simulink model "RobotModel"  (R2020b)
settings: Solver=ode23s  StartTime=tSim(1)  StopTime=tSim(end)  FixedStep=tStep  RelTol=1e-3  EnableMultiTasking=on
values from neighbouring files (symbols this model uses):
  A = [0,0,0,1,0,0;0,0,0,0,1,0;0,0,0,0,0,1;0,981/2480,0,-27/3100,0,0;0,0,-1635,0,0,0;0,-42183/6200,0,9/1550,0,0]    [DeriveCoefficients.m]    (also in InitController.m; SystemAnalysis.m = subs(A_,{phi,z,xd,phid,zd},{0,0,0,0,0}))
  B = [0,0;0,0;0,0;37500/1271,0;0,10000/3;-25000/1271,0]    [DeriveCoefficients.m]    (also in InitController.m; SystemAnalysis.m = subs(B_,{phi,z,xd,phid,zd},{0,0,0,0,0}))
  C = [1,0,0,0,0,0;0,1,0,0,0,0;0,0,1,0,0,0]    [DeriveCoefficients.m]    (also in InitController.m; SystemAnalysis.m = subs(C_,{phi,z,xd,phid,zd},{0,0,0,0,0}))
  Disturbance = 0.1    [SimulateRobot.m]
  g = 9.81    [SimulateRobot.m]    (also in SystemAnalysis.m)
  IC = [xStart; phiStart; zStart; x_dotStart; phi_dotStart; z_dotStart]    [SimulateRobot.m]
  k_r = 7.2e-3    (= 0.0072)    [SimulateRobot.m]
  L = L'    [InitController.m]
  l_S = 5    [SimulateRobot.m]
  l_W = 0.6    [SimulateRobot.m]
  m_B = 0.05    [SimulateRobot.m]
  m_R = 0.8    [SimulateRobot.m]
  m_W = 0.01    [SimulateRobot.m]
  P_max = wM_max*M_max    (= 3.56)    [SimulateRobot.m]
  phi_max = pi/2    (= 1.57079632679)    [SimulateRobot.m]
  r_R = 0.041    [SimulateRobot.m]
  ricatti_controller = lqr(A,B,Q,S)    [InitController.m]
  u_max = 100    [SimulateRobot.m]
  xStart = 0.25    [SimulateRobot.m]
libraries: simulink x1
settings Model: Creator=loehning  LastModifiedBy=klaus
settings DataIOCC: SaveFormat=Array  SignalLoggingSaveFormat=ModelDataLogs  ReturnWorkspaceOutputs=off
settings OptimizationCC: ExpressionDepthLimit=2147483647  LifeSpan=inf
settings DebuggingCC: UnderspecifiedInitializationDetection=Classic  MergeDetectMultiDrivingBlocksExec=none  SolverPrmCheckMsg=warning  FcnCallInpInsideContextMsg=warning  StateNameClashWarn=warning  PregeneratedLibrarySubsystemCodeDiagnostic=none  SFUnexpectedBacktrackingDiag=warning  SFNoUnconditionalDefaultTransitionDiag=warning  SFExecutionAtInitializationDiag=none  ArithmeticOperatorsInVariantConditions=warning
settings HardwareCC: ProdBitPerPointer=32  ProdBitPerSizeT=32  ProdBitPerPtrDiffT=32  ProdLargestAtomicFloat=None  ProdIntDivRoundTo=Undefined  ProdEndianess=Unspecified  ProdWordSize=32  ProdHWDeviceType=32-bit Generic
settings ModelReferenceCC: PropagateSignalLabelsOutOfModel=off
settings SFSimCC: SimUseLocalCustomCode=off  CustomCodeUndefinedFunction=UseInterfaceOnly
settings RTWCC: RTWUseLocalCustomCode=off
settings CodeAppCC: StateflowObjectComments=on
settings GRTTargetCC: TargetLangStandard=C89/C90 (ANSI)  CombineOutputUpdateFcns=off  GRTInterface=on
settings ConfigComp: CovMetricSettings=dw  CovSaveCumulativeToWorkspaceVar=on  CovSaveSingleToWorkspaceVar=on  CovExternalEMLEnable=off  CovSFcnEnable=off

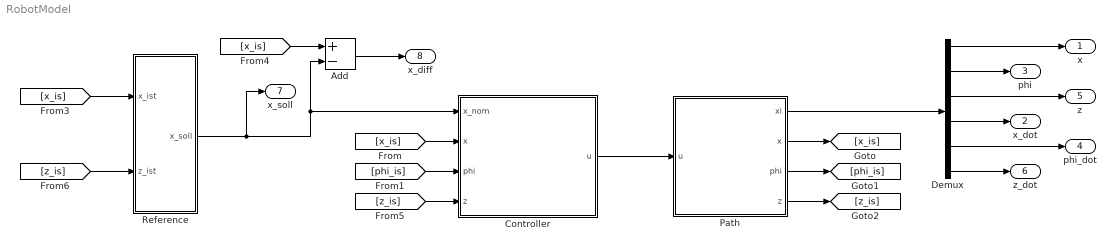
== system RobotModel ==
  Add : Sum  Inputs=+-
  Controller : Subsystem
  Demux : Demux  Outputs=6
  Path : Subsystem
  "Reference " : Subsystem
  x : Outport  VectorParamsAs1DForOutWhenUnconnected=off
  x_dot : Outport  Port=2  VectorParamsAs1DForOutWhenUnconnected=off
  phi : Outport  Port=3  VectorParamsAs1DForOutWhenUnconnected=off
  phi_dot : Outport  Port=4  VectorParamsAs1DForOutWhenUnconnected=off
  z : Outport  Port=5  VectorParamsAs1DForOutWhenUnconnected=off
  z_dot : Outport  Port=6  VectorParamsAs1DForOutWhenUnconnected=off
  x_soll : Outport  Port=7  VectorParamsAs1DForOutWhenUnconnected=off
  x_diff : Outport  Port=8  VectorParamsAs1DForOutWhenUnconnected=off
  wires:
  Path/1(xi) -> Demux/1
  "Reference "/1("x_soll ") -> x_soll/1, Add/2, Controller/1("x_nom ")
  Add/1 -> x_diff/1
  Path/2(x) -> [x_is]
  Path/3(phi) -> [phi_is]
  [x_is] -> Controller/2(x)
  [phi_is] -> Controller/3(phi)
  [z_is] -> "Reference "/2(z_ist)
  [x_is] -> "Reference "/1(x_ist)
  [x_is] -> Add/1
  Path/4(z) -> [z_is]
  [z_is] -> Controller/4(z)
  Demux/1 -> x/1
  Demux/2 -> phi/1
  Demux/3 -> z/1
  Demux/4 -> x_dot/1
  Demux/6 -> z_dot/1
  Demux/5 -> phi_dot/1
  Controller/1(u) -> Path/1("u ")

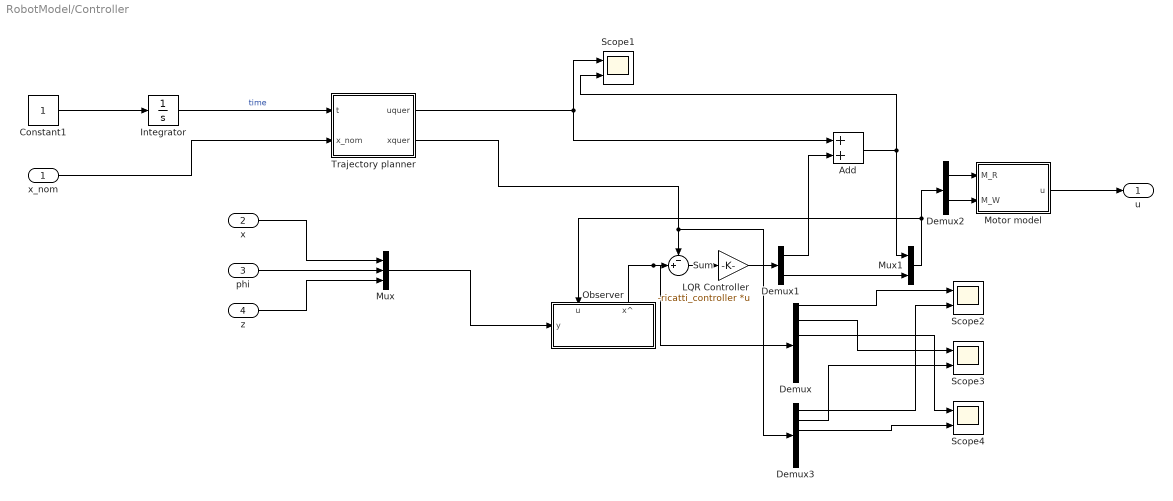
== system RobotModel/Controller ==
  "x_nom " : Inport
  x : Inport  Port=2
  phi : Inport  Port=3
  z : Inport  Port=4
  Add : Sum
  Constant1 : Constant
  Demux : Demux  Outputs=6
  Demux1 : Demux  Outputs=2
  Demux2 : Demux  Outputs=2
  Demux3 : Demux  Outputs=6
  Integrator : Integrator
  LQR Controller : Gain  Gain=-ricatti_controller  Multiplication=Matrix(K*u)
  Motor model : MATLAB Function  TreatAsAtomicUnit=on
  Mux : Mux  Inputs=3
  Mux1 : Mux  Inputs=2
  Observer : Subsystem
      settings: PortSchema="{\"entries\":[{\"content\":{\"sides\":[{\"content\":{\"connectorIds\":[]},\"type\":\"ConnectorPlacement.EquallySpacedRectSide\",\"uuid\":\"22a8423b-4933-4d51-83bb-0edf08131761\"},{\"content\":{\"connectorIds\":[\"In2\"],\"side\":\"RIGHT\"},\"type\":\"ConnectorPlacement.EquallySpacedRectSide\",\"uuid\":\"5b9d6d1b-98ab-4219-9af7-7fee9c92a51b\"},{\"content\":{\"connectorIds\":[],\"side\":\"TOP\"},\"type\":\"ConnectorPlacement.EquallySpacedRectSide\",\"uuid\":\"36e21f0c-31ec-4f4a-8214-47493b03beb7\"},{\"content\":{\"connectorIds\":[\"Out1\",\"In1\"],\"side\":\"BOTTOM\"},\"type\":\"ConnectorPlacement.EquallySpacedRectSide\",\"uuid\":\"16be921e-dd10-4af0-8f26-903c539fc89e\"},{\"content\":{\"connectorIds\":[],\"side\":\"HIDDEN\"},\"type\":\"ConnectorPlacement.EquallySpacedRectSide\",\"uuid\":\"78228177-2ce9-4310-9ad2-dd2810dc3955\"}]},\"type\":\"ConnectorPlacement.EquallySpacedConnector\",\"uuid\":\"efa65d2b-dbcd-4652-bcaa-bff7c8215a9d\"}],\"packageUris\":[\"http://schema.mathworks.com/mf0/Connector/R2020b\"],\"version\":\"1.0\"}"
  Scope{1..4} (4 alike) : Scope  NumInputPorts=2
  Sum : Sum  Inputs=-+|
  Trajectory planner : Subsystem
  u : Outport  VectorParamsAs1DForOutWhenUnconnected=off
  wires:
  Motor model/1(u) -> u/1
  Trajectory planner/1(uquer) -> Scope1/1, Add/1
  Add/1 -> Mux1/1, Scope1/2
  Constant1/1 -> Integrator/1
  Integrator/1 -> Trajectory planner/1(t)  "time"
  Trajectory planner/2(xquer) -> Demux3/1, Sum/1
  "x_nom "/1 -> Trajectory planner/2(x_nom)
  Mux1/1 -> Demux2/1, Observer/1(u)
  phi/1 -> Mux/2
  Mux/1 -> Observer/2(y)
  z/1 -> Mux/3
  x/1 -> Mux/1
  LQR Controller/1 -> Demux1/1
  Demux1/1 -> Add/2
  Demux1/2 -> Mux1/2
  Demux2/1 -> Motor model/1(M_R)
  Demux2/2 -> Motor model/2(M_W)
  Sum/1 -> LQR Controller/1
  Observer/1(x^) -> Demux/1, Sum/2
  Demux/1 -> Scope2/1
  Demux3/1 -> Scope2/2
  Demux/2 -> Scope3/1
  Demux3/2 -> Scope3/2
  Demux/3 -> Scope4/1
  Demux3/3 -> Scope4/2

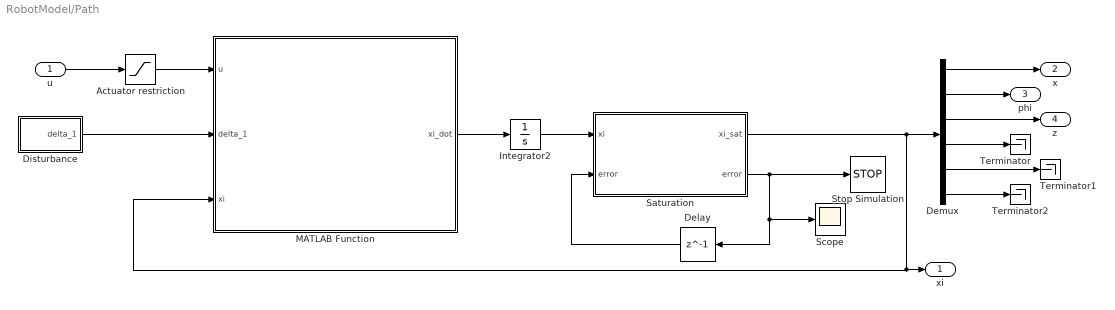
== system RobotModel/Path ==
  "u " : Inport
  Actuator restriction : Saturate  UpperLimit=[u_max;u_max]  LowerLimit=-[u_max;u_max]
  Delay : Delay  DelayLength=1  InitialCondition=0
  Demux : Demux  Outputs=6
  Disturbance : Subsystem
  Integrator2 : Integrator  InitialCondition=IC
  MATLAB Function : MATLAB Function  TreatAsAtomicUnit=on
  "Saturation " : MATLAB Function  TreatAsAtomicUnit=on
  Scope : Scope
  Stop Simulation : Stop
  Terminator : Terminator
  Terminator1 : Terminator
  Terminator2 : Terminator
  xi : Outport  VectorParamsAs1DForOutWhenUnconnected=off
  x : Outport  Port=2  VectorParamsAs1DForOutWhenUnconnected=off
  phi : Outport  Port=3  VectorParamsAs1DForOutWhenUnconnected=off
  z : Outport  Port=4  VectorParamsAs1DForOutWhenUnconnected=off
  wires:
  MATLAB Function/1(xi_dot) -> Integrator2/1
  Delay/1 -> "Saturation "/2("error ")
  "Saturation "/2(error) -> Stop Simulation/1, Scope/1, Delay/1
  Disturbance/1("delta_1 ") -> MATLAB Function/2(delta_1)
  Integrator2/1 -> "Saturation "/1(xi)
  Actuator restriction/1 -> MATLAB Function/1(u)
  Demux/1 -> x/1
  Demux/2 -> phi/1
  Demux/3 -> z/1
  Demux/4 -> Terminator/1
  Demux/5 -> Terminator1/1
  Demux/6 -> Terminator2/1
  "Saturation "/1(xi_sat) -> Demux/1, xi/1, MATLAB Function/3(xi)
  "u "/1 -> Actuator restriction/1

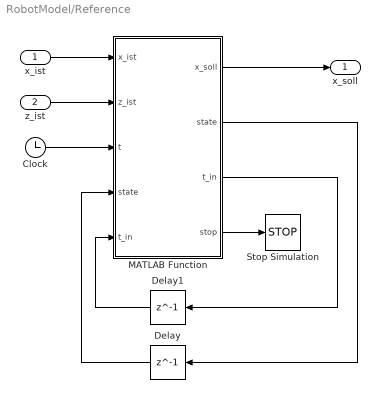
== system RobotModel/Reference  ==
  x_ist : Inport
  z_ist : Inport  Port=2
  Clock : Clock
  Delay : Delay  DelayLength=1  InitialCondition=1
  Delay1 : Delay  DelayLength=1
  MATLAB Function : MATLAB Function  TreatAsAtomicUnit=on
  Stop Simulation : Stop
  "x_soll " : Outport  VectorParamsAs1DForOutWhenUnconnected=off
  wires:
  MATLAB Function/2(state) -> Delay/1
  Delay/1 -> MATLAB Function/4("state ")
  Clock/1 -> MATLAB Function/3(t)
  x_ist/1 -> MATLAB Function/1(x_ist)
  z_ist/1 -> MATLAB Function/2(z_ist)
  MATLAB Function/1(x_soll) -> "x_soll "/1
  MATLAB Function/3(t_in) -> Delay1/1
  Delay1/1 -> MATLAB Function/5("t_in ")
  MATLAB Function/4(stop) -> Stop Simulation/1

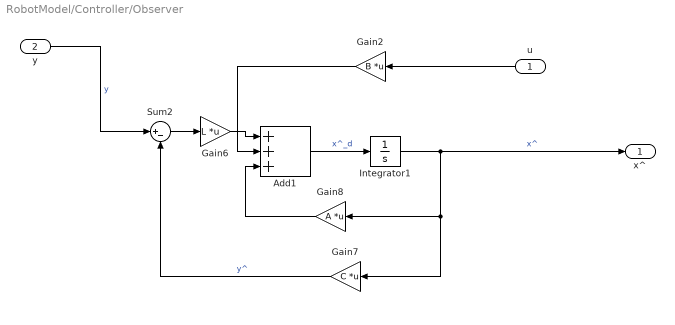
== system RobotModel/Controller/Observer ==
  u : Inport
  y : Inport  Port=2
  Add1 : Sum  Inputs=+++
  Gain2 : Gain  Gain=B  Multiplication=Matrix(K*u)
  Gain6 : Gain  Gain=L  Multiplication=Matrix(K*u)
  Gain7 : Gain  Gain=C  Multiplication=Matrix(K*u)
  Gain8 : Gain  Gain=A  Multiplication=Matrix(K*u)
  Integrator1 : Integrator  InitialCondition=IC
  Sum2 : Sum  Inputs=|+-
  x^ : Outport
  wires:
  Gain2/1 -> Add1/2
  u/1 -> Gain2/1
  Integrator1/1 -> x^/1, Gain7/1, Gain8/1  "x^"
  Gain7/1 -> Sum2/2  "y^"
  y/1 -> Sum2/1  "y"
  Gain6/1 -> Add1/1
  Sum2/1 -> Gain6/1
  Add1/1 -> Integrator1/1  "x^_d"
  Gain8/1 -> Add1/3

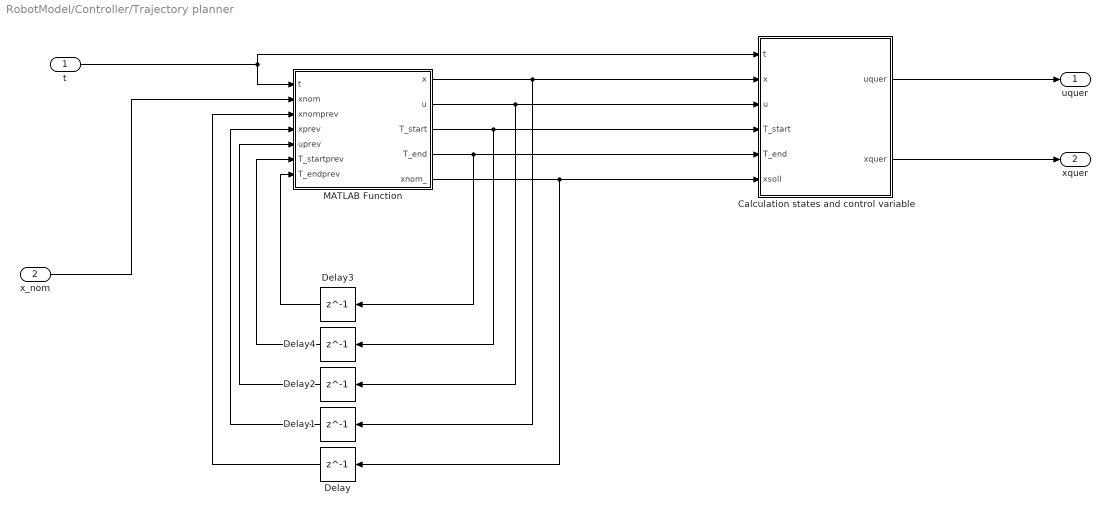
== system RobotModel/Controller/Trajectory planner ==
  t : Inport
  x_nom : Inport  Port=2
  Calculation states and control variable : MATLAB Function  TreatAsAtomicUnit=on
  Delay : Delay  DelayLength=1  InitialCondition=xStart
  Delay{1..4} (4 alike) : Delay  DelayLength=1
  MATLAB Function : MATLAB Function  TreatAsAtomicUnit=on
  uquer : Outport
  xquer : Outport  Port=2
  wires:
  MATLAB Function/1(x) -> Delay1/1, Calculation states and control variable/2(x)
  Delay3/1 -> MATLAB Function/7(T_endprev)
  MATLAB Function/4(T_end) -> Delay3/1, Calculation states and control variable/5(T_end)
  MATLAB Function/2(u) -> Delay2/1, Calculation states and control variable/3(u)
  Delay4/1 -> MATLAB Function/6(T_startprev)
  t/1 -> Calculation states and control variable/1(t), MATLAB Function/1(t)
  Delay1/1 -> MATLAB Function/4(xprev)
  Delay/1 -> MATLAB Function/3(xnomprev)
  MATLAB Function/3(T_start) -> Delay4/1, Calculation states and control variable/4(T_start)
  x_nom/1 -> MATLAB Function/2(xnom)
  Delay2/1 -> MATLAB Function/5(uprev)
  MATLAB Function/5(xnom_) -> Calculation states and control variable/6(xsoll), Delay/1
  Calculation states and control variable/2(xquer) -> xquer/1
  Calculation states and control variable/1(uquer) -> uquer/1

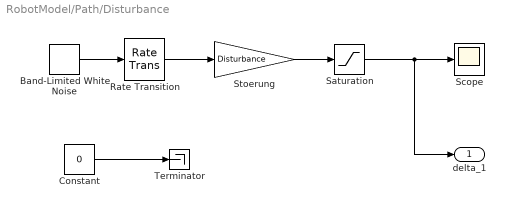
== system RobotModel/Path/Disturbance ==
  Band-Limited White Noise : simulink/Sources/Band-Limited White Noise  Cov=disturbanceNoisePower  Ts=0.025  seed=disturbanceSeed_1
  Constant : Constant  Value=0
  Rate Transition : RateTransition
  Saturation : Saturate  UpperLimit=3  LowerLimit=-3
  Scope : Scope
  Stoerung : Gain  Gain=Disturbance
  Terminator : Terminator
  "delta_1 " : Outport  VectorParamsAs1DForOutWhenUnconnected=off
  wires:
  Band-Limited White Noise/1 -> Rate Transition/1
  Rate Transition/1 -> Stoerung/1
  Stoerung/1 -> Saturation/1
  Saturation/1 -> "delta_1 "/1, Scope/1
  Constant/1 -> Terminator/1

== matlab function RobotModel/Controller/Trajectory planner/Calculation states and control variable ==
  data: t input; uquer output; xquer output; x input; u input; T_start input; T_end input; xsoll input
function [uquer, xquer] = fcn(t, x, u, T_start, T_end, xsoll)
  if t<T_end && size(x,2) == 68 && size(u,2) == 12 
      xquer = [x(1)*(t-T_start)^13+x(2)*(t-T_start)^12+x(3)*(t-T_start)^11+x(4)*(t-T_start)^10+x(5)*(t-T_start)^9+x(6)*(t-T_start)^8+x(7)*(t-T_start)^7+x(8)*(t-T_start)^6+x(9)*(t-T_start)^5+x(10)*(t-T_start)^4+x(11)*(t-T_start)^3+x(12)*(t-T_start)^2+x(13);...
      x(14)*(t-T_start)^12+x(15)*(t-T_start)^11+x(16)*(t-T_start)^10+x(17)*(t-T_start)^9+x(18)*(t-T_start)^8+x(19)*(t-T_start)^7+x(20)*(t-T_start)^6+x(21)*(t-T_start)^5+x(22)*(t-T_start)^4+x(23)*(t-T_start)^3+x(24)*(t-T_start)^2;...
      x(25)*(t-T_start)^12+x(26)*(t-T_start)^11+x(27)*(t-T_start)^10+x(28)*(t-T_start)^9+x(29)*(t-T_start)^8+x(30)*(t-T_start)^7+x(31)*(t-T_start)^6+x(32)*(t-T_start)^5+x(33)*(t-T_start)^4+x(34)*(t-T_start)^3+x(35)*(t-T_start)^2;...
      x(36)*(t-T_start)^12+x(37)*(t-T_start)^11+x(38)*(t-T_start)^10+x(39)*(t-T_start)^9+x(40)*(t-T_start)^8+x(41)*(t-T_start)^7+x(42)*(t-T_start)^6+x(43)*(t-T_start)^5+x(44)*(t-T_start)^4+x(45)*(t-T_start)^3+x(46)*(t-T_start)^2;...
      x(47)*(t-T_start)^12+x(48)*(t-T_start)^11+x(49)*(t-T_start)^10+x(50)*(t-T_start)^9+x(51)*(t-T_start)^8+x(52)*(t-T_start)^7+x(53)*(t-T_start)^6+x(54)*(t-T_start)^5+x(55)*(t-T_start)^4+x(56)*(t-T_start)^3+x(57)*(t-T_start)^2;...
      x(58)*(t-T_start)^12+x(59)*(t-T_start)^11+x(60)*(t-T_start)^10+x(61)*(t-T_start)^9+x(62)*(t-T_start)^8+x(63)*(t-T_start)^7+x(64)*(t-T_start)^6+x(65)*(t-T_start)^5+x(66)*(t-T_start)^4+x(67)*(t-T_start)^3+x(68)*(t-T_start)^2];
      uquer = u(1)*(t-T_start)^12+u(2)*(t-T_start)^11+u(3)*(t-T_start)^10+u(4)*(t-T_start)^9+u(5)*(t-T_start)^8+u(6)*(t-T_start)^7+u(7)*(t-T_start)^6+u(8)*(t-T_start)^5+u(9)*(t-T_start)^4+u(10)*(t-T_start)^3+u(11)*(t-T_start)^2+u(12)*(t-T_start);
  else
      xquer = [xsoll;0;0;0;0;0];      
      uquer = 0;
  end  
end

== matlab function RobotModel/Controller/Trajectory planner/MATLAB Function ==
  data: x output; t input; xnom input; u output; xnomprev input; T_start output; T_end output; xnom_ output; xprev input; uprev input; T_startprev input; T_endprev input
function [x, u, T_start, T_end, xnom_] = fcn(t, xnom, xnomprev, xprev, uprev, T_startprev, T_endprev)
    if xnom ~= xnomprev
        w0 = xnomprev;
        wT = xnom;
        order = [12,11,10,9,8,7,6,5,4,3,2,1];
        T_end = abs(w0-wT)/0.7;
        if T_end<1
            T_end=1;
        end
        u1 = [(1011384551389116279375*(w0 - wT))/(36893488147419103232*T_end^7), (1092295315500245581725*(w0 - wT))/(9149585060559937601536*T_end^7) - (21239075579171441866875*(w0 - wT))/(36893488147419103232*T_end^8), (35398459298619069778125*(w0 - wT))/(9223372036854775808*T_end^9) - (7646067208501719072075*(w0 - wT))/(4574792530279968800768*T_end^8) - (142538111831879000698793027470149375*(w0 - wT))/(6901746346790563787434755862277025452451108972170386555162524223799296*T_end^7), (2993300348469459014674653576873136875*(w0 - wT))/(13803492693581127574869511724554050904902217944340773110325048447598592*T_end^8) + (38230336042508595360375*(w0 - wT))/(4574792530279968800768*T_end^9) - (106195377895857209334375*(w0 - wT))/(9223372036854775808*T_end^10), (318586133687571628003125*(w0 - wT))/(18446744073709551616*T_end^11) - (2993300348469459014674653576873136875*(w0 - wT))/(3450873173395281893717377931138512726225554486085193277581262111899648*T_end^9) - (22938201625505157216225*(w0 - wT))/(1143698132569992200192*T_end^10) - (51542850267891542935087149177365625*(w0 - wT))/(20282409603651670423947251286016*T_end^7), (360799951875240800545610044241559375*(w0 - wT))/(20282409603651670423947251286016*T_end^8) - (36823171168130880507853335496664625*(w0 - wT))/(10384593717069655257060992658440192*T_end^7) + (2993300348469459014674653576873136875*(w0 - wT))/(1725436586697640946858688965569256363112777243042596638790631055949824*T_end^10) + (114691008127525786081125*(w0 - wT))/(4574792530279968800768*T_end^11) - (233629831370885860535625*(w0 - wT))/(18446744073709551616*T_end^12), (110469513504392641523560006489993875*(w0 - wT))/(5192296858534827628530496329220096*T_end^8) - (257714251339457714675435745886828125*(w0 - wT))/(5070602400912917605986812821504*T_end^9) - (6414215032434555031445686236156721875*(w0 - wT))/(3450873173395281893717377931138512726225554486085193277581262111899648*T_end^11) - (36045745411508104196925*(w0 - wT))/(2287396265139984400384*T_end^12) + (33375690195840837219375*(w0 - wT))/(9223372036854775808*T_end^13), (773142754018373144026307237660484375*(w0 - wT))/(10141204801825835211973625643008*T_end^10) - (552347567521963207617800032449969375*(w0 - wT))/(10384593717069655257060992658440192*T_end^9) + (14111273071356021069180509719544788125*(w0 - wT))/(13803492693581127574869511724554050904902217944340773110325048447598592*T_end^12) + (36045745411508104196925*(w0 - wT))/(9149585060559937601536*T_end^13), (184115855840654402539266677483323125*(w0 - wT))/(2596148429267413814265248164610048*T_end^10) - (1288571256697288573377178729434140625*(w0 - wT))/(20282409603651670423947251286016*T_end^11) - (1567919230150669007686723302171643125*(w0 - wT))/(6901746346790563787434755862277025452451108972170386555162524223799296*T_end^13), (566971352946806972285958640951021875*(w0 - wT))/(20282409603651670423947251286016*T_end^12) - (552347567521963207617800032449969375*(w0 - wT))/(10384593717069655257060992658440192*T_end^11), (110469513504392641523560006489993875*(w0 - wT))/(5192296858534827628530496329220096*T_end^12) - (51542850267891542935087149177365625*(w0 - wT))/(10141204801825835211973625643008*T_end^13), -(36823171168130880507853335496664625*(w0 - wT))/(10384593717069655257060992658440192*T_end^13)];
        u = double(u1(order));
        order = [13,12,11,10,9,8,7,6,5,4,3,2,1,24,23,22,21,20,19,18,17,16,15,14,35,34,33,32,31,30,29,28,27,26,25,46,45,44,43,42,41,40,39,38,37,36,57,56,55,54,53,52,51,50,49,48,47,68,67,66,65,64,63,62,61,60,59,58];
        x1 = [w0, -(91300322845796259195*(w0 - wT))/(89202980794122492566142873090593446023921664*T_end^7), (155417816831775633135*(w0 - wT))/(1152921504606846976*T_end^7) + (639102259920573814365*(w0 - wT))/(44601490397061246283071436545296723011960832*T_end^8), - (159970356708403816575*(w0 - wT))/(340282366920938463463374607431768211456*T_end^7) - (3263774153467288295835*(w0 - wT))/(2305843009213693952*T_end^8) - (3195511299602869071825*(w0 - wT))/(44601490397061246283071436545296723011960832*T_end^9), (15686105019335663913*(w0 - wT))/(43556142965880123323311949751266331066368*T_end^7) + (671875498175296029615*(w0 - wT))/(170141183460469231731687303715884105728*T_end^8) + (3263774153467288295835*(w0 - wT))/(576460752303423488*T_end^9) + (1917306779761721443095*(w0 - wT))/(11150372599265311570767859136324180752990208*T_end^10), (21186311244744238593*(w0 - wT))/(696898287454081973172991196020261297061888*T_end^7) - (109802735135349647391*(w0 - wT))/(43556142965880123323311949751266331066368*T_end^8) - (1119792496958826716025*(w0 - wT))/(85070591730234615865843651857942052864*T_end^9) - (3263774153467288295835*(w0 - wT))/(288230376151711744*T_end^10) - (9586533898808607215475*(w0 - wT))/(44601490397061246283071436545296723011960832*T_end^11), (78430525096678319565*(w0 - wT))/(10889035741470030830827987437816582766592*T_end^9) - (63558933734232715779*(w0 - wT))/(348449143727040986586495598010130648530944*T_end^8) - (1716*(w0 - wT))/T_end^7 + (479911070125211449725*(w0 - wT))/(21267647932558653966460912964485513216*T_end^10) + (6993801757429903491075*(w0 - wT))/(576460752303423488*T_end^11) + (3012910653911276553435*(w0 - wT))/(22300745198530623141535718272648361505980416*T_end^12), (9009*(w0 - wT))/T_end^8 + (317794668671163578895*(w0 - wT))/(696898287454081973172991196020261297061888*T_end^9) - (235291575290034958695*(w0 - wT))/(21778071482940061661655974875633165533184*T_end^10) - (7198666051878171745875*(w0 - wT))/(340282366920938463463374607431768211456*T_end^11) - (15386363866345787680365*(w0 - wT))/(2305843009213693952*T_end^12) - (3012910653911276553435*(w0 - wT))/(89202980794122492566142873090593446023921664*T_end^13), (392152625483391597825*(w0 - wT))/(43556142965880123323311949751266331066368*T_end^11) - (105931556223721192965*(w0 - wT))/(174224571863520493293247799005065324265472*T_end^10) - (20020*(w0 - wT))/T_end^9 + (1759673923792441982325*(w0 - wT))/(170141183460469231731687303715884105728*T_end^12) + (1709595985149531964485*(w0 - wT))/(1152921504606846976*T_end^13), (24024*(w0 - wT))/T_end^10 + (317794668671163578895*(w0 - wT))/(696898287454081973172991196020261297061888*T_end^11) - (172547155212692303043*(w0 - wT))/(43556142965880123323311949751266331066368*T_end^12) - (351934784758488396465*(w0 - wT))/(170141183460469231731687303715884105728*T_end^13), (15686105019335663913*(w0 - wT))/(21778071482940061661655974875633165533184*T_end^13) - (63558933734232715779*(w0 - wT))/(348449143727040986586495598010130648530944*T_end^12) - (16380*(w0 - wT))/T_end^11, (6006*(w0 - wT))/T_end^12 + (21186311244744238593*(w0 - wT))/(696898287454081973172991196020261297061888*T_end^13), -(924*(w0 - wT))/T_end^13, -(1213230839868007845885*(w0 - wT))/(85070591730234615865843651857942052864*T_end^7), (8492615879076054921195*(w0 - wT))/(42535295865117307932921825928971026432*T_end^8) - (252577308855890773755*(w0 - wT))/(10889035741470030830827987437816582766592*T_end^7), (5304123485973706248855*(w0 - wT))/(21778071482940061661655974875633165533184*T_end^8) - (74318744670378353145*(w0 - wT))/(1393796574908163946345982392040522594123776*T_end^7) - (42463079395380274605975*(w0 - wT))/(42535295865117307932921825928971026432*T_end^9), (800800*(w0 - wT))/(109*T_end^7) + (312138727615589083209*(w0 - wT))/(696898287454081973172991196020261297061888*T_end^8) - (5304123485973706248855*(w0 - wT))/(5444517870735015415413993718908291383296*T_end^9) + (25477847637228164763585*(w0 - wT))/(10633823966279326983230456482242756608*T_end^10), (5304123485973706248855*(w0 - wT))/(2722258935367507707706996859454145691648*T_end^10) - (5605600*(w0 - wT))/(109*T_end^8) - (520231212692648472015*(w0 - wT))/(348449143727040986586495598010130648530944*T_end^9) - (22057997440968149661*(w0 - wT))/(5192296858534827628530496329220096*T_end^7) - (127389238186140823817925*(w0 - wT))/(42535295865117307932921825928971026432*T_end^11), (66173992322904448983*(w0 - wT))/(2596148429267413814265248164610048*T_end^8) + (16016000*(w0 - wT))/(109*T_end^9) + (222956234011135059435*(w0 - wT))/(87112285931760246646623899502532662132736*T_end^10) - (11365978898515084818975*(w0 - wT))/(5444517870735015415413993718908291383296*T_end^11) + (40036617715644258914205*(w0 - wT))/(21267647932558653966460912964485513216*T_end^12), (25005153576733186601745*(w0 - wT))/(21778071482940061661655974875633165533184*T_end^12) - (24024000*(w0 - wT))/(109*T_end^10) - (3344343510167025891525*(w0 - wT))/(1393796574908163946345982392040522594123776*T_end^11) - (330869961614522244915*(w0 - wT))/(5192296858534827628530496329220096*T_end^9) - (40036617715644258914205*(w0 - wT))/(85070591730234615865843651857942052864*T_end^13), (110289987204840748305*(w0 - wT))/(1298074214633706907132624082305024*T_end^10) + (20020000*(w0 - wT))/(109*T_end^11) + (817506191374161884595*(w0 - wT))/(696898287454081973172991196020261297061888*T_end^12) - (2778350397414798511305*(w0 - wT))/(10889035741470030830827987437816582766592*T_end^13), - (330869961614522244915*(w0 - wT))/(5192296858534827628530496329220096*T_end^11) - (8808800*(w0 - wT))/(109*T_end^12) - (163501238274832376919*(w0 - wT))/(696898287454081973172991196020261297061888*T_end^13), (66173992322904448983*(w0 - wT))/(2596148429267413814265248164610048*T_end^12) + (1601600*(w0 - wT))/(109*T_end^13), -(22057997440968149661*(w0 - wT))/(5192296858534827628530496329220096*T_end^13), (486935055177579913905*(w0 - wT))/(713623846352979940529142984724747568191373312*T_end^7), - (25902969471962598015*(w0 - wT))/(288230376151711744*T_end^7) - (3408545386243059397335*(w0 - wT))/(356811923176489970264571492362373784095686656*T_end^8), (228719772458392380165*(w0 - wT))/(2658455991569831745807614120560689152*T_end^7) + (543962358911214558315*(w0 - wT))/(576460752303423488*T_end^8) + (17042726931215296986675*(w0 - wT))/(356811923176489970264571492362373784095686656*T_end^9), (79978429159320330639*(w0 - wT))/(10889035741470030830827987437816582766592*T_end^7) - (960623044325247996693*(w0 - wT))/(1329227995784915872903807060280344576*T_end^8) - (543962358911214558315*(w0 - wT))/(144115188075855872*T_end^9) - (10225636158729178192005*(w0 - wT))/(89202980794122492566142873090593446023921664*T_end^10), (1601038407208746661155*(w0 - wT))/(664613997892457936451903530140172288*T_end^9) - (559849004115242314473*(w0 - wT))/(10889035741470030830827987437816582766592*T_end^8) - (12046928654849835747*(w0 - wT))/(1393796574908163946345982392040522594123776*T_end^7) + (543962358911214558315*(w0 - wT))/(72057594037927936*T_end^10) + (51128180793645890960025*(w0 - wT))/(356811923176489970264571492362373784095686656*T_end^11), (36140785964549507241*(w0 - wT))/(696898287454081973172991196020261297061888*T_end^8) + (399892145796601653195*(w0 - wT))/(2722258935367507707706996859454145691648*T_end^9) - (686159317375177140495*(w0 - wT))/(166153499473114484112975882535043072*T_end^10) - (1165633626238316910675*(w0 - wT))/(144115188075855872*T_end^11) - (16068856820860137158865*(w0 - wT))/(178405961588244985132285746181186892047843328*T_end^12), (10292389760627657107425*(w0 - wT))/(2658455991569831745807614120560689152*T_end^11) - (1199676437389804959585*(w0 - wT))/(5444517870735015415413993718908291383296*T_end^10) - (180703929822747536205*(w0 - wT))/(1393796574908163946345982392040522594123776*T_end^9) + (2564393977724297203485*(w0 - wT))/(576460752303423488*T_end^12) + (16068856820860137158865*(w0 - wT))/(713623846352979940529142984724747568191373312*T_end^13), (60234643274249178735*(w0 - wT))/(348449143727040986586495598010130648530944*T_end^10) + (1999460728983008265975*(w0 - wT))/(10889035741470030830827987437816582766592*T_end^11) - (2515917497042316181815*(w0 - wT))/(1329227995784915872903807060280344576*T_end^12) - (284932664191588578165*(w0 - wT))/(288230376151711744*T_end^13), (503183499408463236363*(w0 - wT))/(1329227995784915872903807060280344576*T_end^13) - (879762720752523637029*(w0 - wT))/(10889035741470030830827987437816582766592*T_end^12) - (180703929822747536205*(w0 - wT))/(1393796574908163946345982392040522594123776*T_end^11), (36140785964549507241*(w0 - wT))/(696898287454081973172991196020261297061888*T_end^12) + (79978429159320330639*(w0 - wT))/(5444517870735015415413993718908291383296*T_end^13), -(12046928654849835747*(w0 - wT))/(1393796574908163946345982392040522594123776*T_end^13), (466253450495326899405*(w0 - wT))/(1152921504606846976*T_end^7), - (319940713416817227735*(w0 - wT))/(170141183460469231731687303715884105728*T_end^7) - (3263774153467288295835*(w0 - wT))/(576460752303423488*T_end^8), (313722100386713683665*(w0 - wT))/(174224571863520493293247799005065324265472*T_end^7) + (6718754981753161782435*(w0 - wT))/(340282366920938463463374607431768211456*T_end^8) + (16318870767336441479175*(w0 - wT))/(576460752303423488*T_end^9), - (41005763699505051447*(w0 - wT))/(5575186299632655785383929568162090376495104*T_end^7) - (1317632821624197471393*(w0 - wT))/(87112285931760246646623899502532662132736*T_end^8) - (6718754981753161782435*(w0 - wT))/(85070591730234615865843651857942052864*T_end^9) - (9791322460401864887505*(w0 - wT))/(144115188075855872*T_end^10), (287040345896535360129*(w0 - wT))/(5575186299632655785383929568162090376495104*T_end^8) - (12012*(w0 - wT))/T_end^7 + (2196054702706995785655*(w0 - wT))/(43556142965880123323311949751266331066368*T_end^9) + (6718754981753161782435*(w0 - wT))/(42535295865117307932921825928971026432*T_end^10) + (48956612302009324437525*(w0 - wT))/(576460752303423488*T_end^11), (72072*(w0 - wT))/T_end^8 - (205028818497525257235*(w0 - wT))/(1393796574908163946345982392040522594123776*T_end^9) - (941166301160141050995*(w0 - wT))/(10889035741470030830827987437816582766592*T_end^10) - (14397332103756775248075*(w0 - wT))/(85070591730234615865843651857942052864*T_end^11) - (15386363866345787680365*(w0 - wT))/(288230376151711744*T_end^12), (615086455492575771705*(w0 - wT))/(2787593149816327892691964784081045188247552*T_end^10) - (180180*(w0 - wT))/T_end^9 + (14117494517402115764925*(w0 - wT))/(174224571863520493293247799005065324265472*T_end^11) + (31674130628264905545765*(w0 - wT))/(340282366920938463463374607431768211456*T_end^12) + (15386363866345787680365*(w0 - wT))/(1152921504606846976*T_end^13), (240240*(w0 - wT))/T_end^10 - (1025144092487626286175*(w0 - wT))/(5575186299632655785383929568162090376495104*T_end^11) - (3450943104253850520315*(w0 - wT))/(87112285931760246646623899502532662132736*T_end^12) - (3519347847584989505085*(w0 - wT))/(170141183460469231731687303715884105728*T_end^13), (451063400694555565917*(w0 - wT))/(5575186299632655785383929568162090376495104*T_end^12) - (180180*(w0 - wT))/T_end^11 + (690188620850770104063*(w0 - wT))/(87112285931760246646623899502532662132736*T_end^13), (72072*(w0 - wT))/T_end^12 - (41005763699505051447*(w0 - wT))/(2787593149816327892691964784081045188247552*T_end^13), -(12012*(w0 - wT))/T_end^13, (594824777491629980295*(w0 - wT))/(10889035741470030830827987437816582766592*T_end^7), - (297274978681513457625*(w0 - wT))/(1393796574908163946345982392040522594123776*T_end^7) - (4163773442441409862065*(w0 - wT))/(5444517870735015415413993718908291383296*T_end^8), (4004000*(w0 - wT))/(109*T_end^7) + (6242774552311782610125*(w0 - wT))/(2787593149816327892691964784081045188247552*T_end^8) + (20818867212207049310325*(w0 - wT))/(5444517870735015415413993718908291383296*T_end^9), - (36519221481393702051*(w0 - wT))/(1298074214633706907132624082305024*T_end^7) - (33633600*(w0 - wT))/(109*T_end^8) - (6242774552311782610125*(w0 - wT))/(696898287454081973172991196020261297061888*T_end^9) - (12491320327324229586195*(w0 - wT))/(1361129467683753853853498429727072845824*T_end^10), (255634550369755914357*(w0 - wT))/(1298074214633706907132624082305024*T_end^8) - (19616364991367881737*(w0 - wT))/(5316911983139663491615228241121378304*T_end^7) + (112112000*(w0 - wT))/(109*T_end^9) + (6242774552311782610125*(w0 - wT))/(348449143727040986586495598010130648530944*T_end^10) + (62456601636621147930975*(w0 - wT))/(5444517870735015415413993718908291383296*T_end^11), (58849094974103645211*(w0 - wT))/(2658455991569831745807614120560689152*T_end^8) - (182596107406968510255*(w0 - wT))/(324518553658426726783156020576256*T_end^9) - (192192000*(w0 - wT))/(109*T_end^10) - (13377374040668105593125*(w0 - wT))/(696898287454081973172991196020261297061888*T_end^11) - (19629217657223789349735*(w0 - wT))/(2722258935367507707706996859454145691648*T_end^12), (547788322220905530765*(w0 - wT))/(649037107316853453566312041152512*T_end^10) - (294245474870518226055*(w0 - wT))/(5316911983139663491615228241121378304*T_end^9) + (180180000*(w0 - wT))/(109*T_end^11) + (29430222889469832304875*(w0 - wT))/(2787593149816327892691964784081045188247552*T_end^12) + (19629217657223789349735*(w0 - wT))/(10889035741470030830827987437816582766592*T_end^13), (98081824956839408685*(w0 - wT))/(1329227995784915872903807060280344576*T_end^10) - (912980537034842551275*(w0 - wT))/(1298074214633706907132624082305024*T_end^11) - (88088000*(w0 - wT))/(109*T_end^12) - (3270024765496648033875*(w0 - wT))/(1393796574908163946345982392040522594123776*T_end^13), (401711436295330722561*(w0 - wT))/(1298074214633706907132624082305024*T_end^12) - (294245474870518226055*(w0 - wT))/(5316911983139663491615228241121378304*T_end^11) + (17617600*(w0 - wT))/(109*T_end^13), (58849094974103645211*(w0 - wT))/(2658455991569831745807614120560689152*T_end^12) - (36519221481393702051*(w0 - wT))/(649037107316853453566312041152512*T_end^13), -(19616364991367881737*(w0 - wT))/(5316911983139663491615228241121378304*T_end^13), -(77708908415887794045*(w0 - wT))/(288230376151711744*T_end^7), (114359886229196212605*(w0 - wT))/(332306998946228968225951765070086144*T_end^7) + (543962358911214558315*(w0 - wT))/(144115188075855872*T_end^8), (199946072898300804075*(w0 - wT))/(5444517870735015415413993718908291383296*T_end^7) - (2401557610813120464705*(w0 - wT))/(664613997892457936451903530140172288*T_end^8) - (2719811794556072791575*(w0 - wT))/(144115188075855872*T_end^9), (52021605989386196163*(w0 - wT))/(696898287454081973172991196020261297061888*T_end^7) - (839773506172863377115*(w0 - wT))/(2722258935367507707706996859454145691648*T_end^8) + (2401557610813120464705*(w0 - wT))/(166153499473114484112975882535043072*T_end^9) + (1631887076733643674945*(w0 - wT))/(36028797018963968*T_end^10), (15746213260609909077*(w0 - wT))/(89202980794122492566142873090593446023921664*T_end^7) - (364151241925703373141*(w0 - wT))/(696898287454081973172991196020261297061888*T_end^8) + (1399622510288105628525*(w0 - wT))/(1361129467683753853853498429727072845824*T_end^9) - (2401557610813120464705*(w0 - wT))/(83076749736557242056487941267521536*T_end^10) - (8159435383668218374725*(w0 - wT))/(144115188075855872*T_end^11), (260108029946930980815*(w0 - wT))/(174224571863520493293247799005065324265472*T_end^9) - (47238639781829727231*(w0 - wT))/(44601490397061246283071436545296723011960832*T_end^8) - (599838218694902412225*(w0 - wT))/(340282366920938463463374607431768211456*T_end^10) + (5146194880313829567225*(w0 - wT))/(166153499473114484112975882535043072*T_end^11) + (2564393977724297203485*(w0 - wT))/(72057594037927936*T_end^12), (236193198909148636155*(w0 - wT))/(89202980794122492566142873090593446023921664*T_end^9) - (780324089840792942445*(w0 - wT))/(348449143727040986586495598010130648530944*T_end^10) + (8997573280423536183375*(w0 - wT))/(5444517870735015415413993718908291383296*T_end^11) - (11321628736690425047895*(w0 - wT))/(664613997892457936451903530140172288*T_end^12) - (2564393977724297203485*(w0 - wT))/(288230376151711744*T_end^13), (1300540149734654904075*(w0 - wT))/(696898287454081973172991196020261297061888*T_end^11) - (78731066303049545385*(w0 - wT))/(22300745198530623141535718272648361505980416*T_end^10) - (2199406801881308844825*(w0 - wT))/(2722258935367507707706996859454145691648*T_end^12) + (1257958748521158338655*(w0 - wT))/(332306998946228968225951765070086144*T_end^13), (236193198909148636155*(w0 - wT))/(89202980794122492566142873090593446023921664*T_end^11) - (572237665883248157793*(w0 - wT))/(696898287454081973172991196020261297061888*T_end^12) + (439881360376261768965*(w0 - wT))/(2722258935367507707706996859454145691648*T_end^13), (52021605989386196163*(w0 - wT))/(348449143727040986586495598010130648530944*T_end^13) - (47238639781829727231*(w0 - wT))/(44601490397061246283071436545296723011960832*T_end^12), (15746213260609909077*(w0 - wT))/(89202980794122492566142873090593446023921664*T_end^13)];
        x = double(x1(order));
        T_start = t;
        T_end = t+T_end;
        xnom_ = xnom;
    else
        x = xprev;
        u = uprev;
        T_start = T_startprev;
        T_end = T_endprev;
        xnom_ = xnom;
    end
end

== matlab function RobotModel/Path/MATLAB Function ==
  data: u input; delta_1 input; xi_dot output size=[6 1]; xi input size=[6 1]; m_B parameter; m_R parameter; r_R parameter; l_W parameter; m_W parameter; g parameter; k_r parameter; P_max parameter; u_max parameter
function xi_dot   = pathDynamic(u, delta_1, xi, m_B, m_R, r_R, l_W, m_W, g, k_r, P_max, u_max)

% Robot, beam and ball dynamics

% Motor torque robot
u_R = u(1);
P_R = (u_R+delta_1)/u_max*P_max; %Engine power
M_R_max = sqrt(abs(P_R))/9.434;

M_R = 2*sign2(u_R+delta_1)*M_R_max; % Total torque

% Motor torque beam
u_W =  u(2);
P_W = (u_W+delta_1)/u_max*P_max;
M_W_max = sqrt(abs(P_W))/9.434;

M_W = sign2(u_W+delta_1)*M_W_max;

nu = [M_R; M_W];

% Equations of motion
xi_dot = statespace_model(m_B, m_R, r_R, l_W, m_W, g, k_r, xi, nu);

end
function outp =  sign2(inp)
    if(inp == 0) 
        outp = -1;
    else
        outp = sign(inp);
    end
end

== matlab function RobotModel/Reference /MATLAB Function ==
  data: x_ist input; x_soll output; z_ist input; t input; state input; state output; t_in input; t_in output; stop output
function [x_soll,state,t_in,stop] = reference(x_ist,z_ist,t,state,t_in)
x_bound = 20*10^-3;
z_bound = 20*10^-3;
t_bound = 1.5;
stop = 0;

%y_ref_vec = [0.2,-2,-1,-2.4,0,0.1,0.2,2,0];
y_ref_vec = [0.2,-0,-0.5,-1.5,-2.4,-1.5,-1,0];
if(state <= size(y_ref_vec,2))
    x_soll = y_ref_vec(state);
    if(abs(x_ist-y_ref_vec(state)) > x_bound)
        t_in = t;
    end
    if(abs(z_ist-0) > z_bound)
        t_in = t;
    end
    if(t-t_in > t_bound)
        state = state+1;
        t_in = t;
    end
    
else
    x_soll = y_ref_vec(size(y_ref_vec,2));
    stop = 1;
end

== matlab function RobotModel/Path/Saturation  ==
  data: xi input size=[6 1]; error input; phi_max parameter; xi_sat output size=[6 1]; l_S parameter; error output; l_W parameter
function [xi_sat,error]  = fcn(xi, error, phi_max, l_S, l_W)

xi_sat = xi;

% Saturation in y
if xi(1) >= l_S/2
    xi_sat(1) = l_S/2;
    xi_sat(4) = 0; % Roboter fällt herunter!!!!
    error = 1;
end

if xi(1) <= -l_S/2
    xi_sat(1) = -l_S/2;
    xi_sat(4) = 0; % Roboter fällt herunter!!!!
    error = 1;
end

% Saturation in phi
if (abs(xi(2)) > phi_max) 
    error = 1; % Ball verliert Kontakt mit Wippe!!!
end

% Saturation in z

if xi(3) >= l_W/2
    xi_sat(3) = l_W/2;
    xi_sat(6) = 0; % Ball fällt herunter!!!!
    error = 1;
end

if xi(3) <= -l_W/2
    xi_sat(3) = -l_W/2;
    xi_sat(6) = 0; % Ball fällt herunter!!!!
    error = 1;
end

% error-Schleife

if (error)
    xi_sat = zeros(6,1);
end

== matlab function RobotModel/Controller/Motor model ==
  data: M_R input; u output; M_W input
function u = fcn(M_R,M_W)
    invertM_R = 0;
    invertM_W = 0;
    if M_R<0
        invertM_R=1;
    end
    if M_W<0
        invertM_W=1;
    end
    u_R_solved = (250001*M_R^2)/400;
    u_W_solved = (250001*M_W^2)/100;
    if invertM_R==1
        u_R_solved=u_R_solved*(-1);
    end
    if invertM_W==1
        u_W_solved=u_W_solved*(-1);
    end

    u = [u_R_solved; u_W_solved]; 
end
